simulink model "lab2"  (R2024a)
settings: Solver=FixedStepAuto  StartTime=0.0  StopTime=10.0  FixedStep=0.01  RelTol=1e-3
settings Model: Creator=ventus  LastModifiedBy=ventus

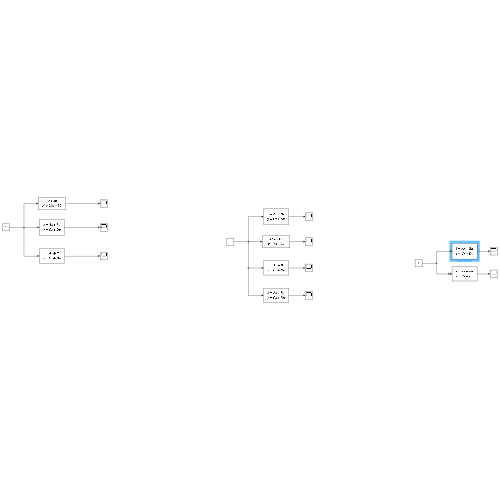
[thumbnail: Simulink's stored preview of the top-level diagram]
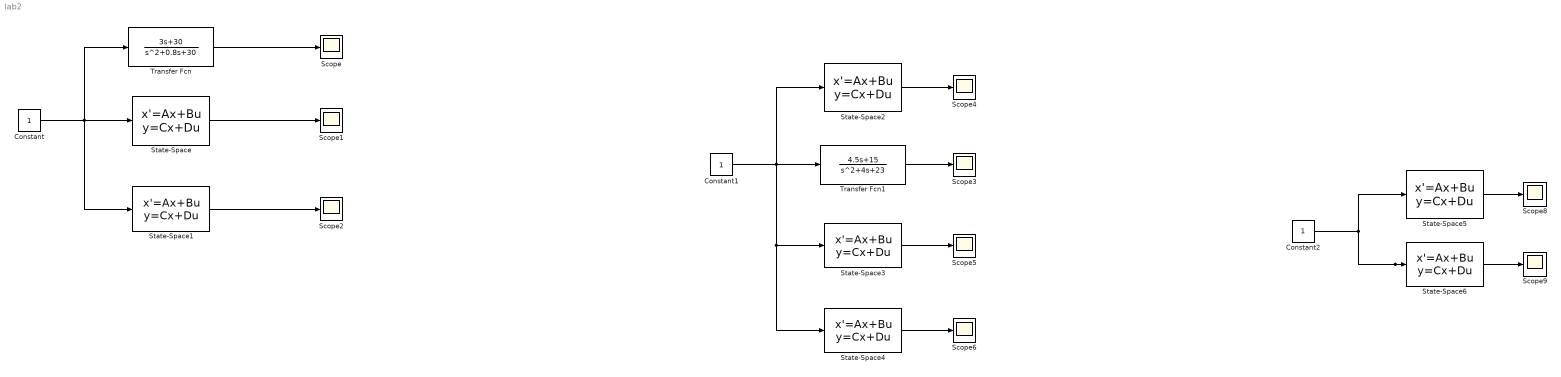
== system lab2 ==
  Constant : Constant
  Constant1 : Constant
  Constant2 : Constant
  Scope{,1..6,8..9} (9 alike) : Scope
  State-Space : StateSpace  A=[0 1; -30 -0.8]  B=[0; 1]  C=[30 3]  D=0  InitialCondition=0
  State-Space1 : StateSpace  A=[0 -30; 1 -0.8]  B=[30; 3]  C=[0 1]  D=0  InitialCondition=0
  State-Space2 : StateSpace  A=[-1 2; -10 -3]  B=[0.5; 1]  C=[6 1.5]  D=0  InitialCondition=0
  State-Space3 : StateSpace  A=[0 1; -23 -4]  B=[0; 1]  C=[15 4.5]  D=0  InitialCondition=0
  State-Space4 : StateSpace  A=[0 -23; 1 -4]  B=[15; 4.5]  C=[0 1]  D=0  InitialCondition=0
  State-Space5 : StateSpace  A=[-1 2; -10 -3]  B=[0.5; 1]  C=[6.5 1.5]  D=0  InitialCondition=0
  State-Space6 : StateSpace  A=[9 28; -5 -13]  B=[-0.5; 0.5]  C=[6.5 16]  D=0  InitialCondition=0
  Transfer Fcn : TransferFcn  Numerator=[3 30]  Denominator=[1 0.8 30]
  Transfer Fcn1 : TransferFcn  Numerator=[4.5 15]  Denominator=[1 4 23]
  wires:
  Constant/1 -> Transfer Fcn/1, State-Space/1, State-Space1/1
  State-Space/1 -> Scope1/1
  Transfer Fcn/1 -> Scope/1
  State-Space1/1 -> Scope2/1
  State-Space3/1 -> Scope5/1
  Transfer Fcn1/1 -> Scope3/1
  Constant1/1 -> State-Space4/1, State-Space3/1, State-Space2/1, Transfer Fcn1/1
  State-Space2/1 -> Scope4/1
  State-Space4/1 -> Scope6/1
  State-Space5/1 -> Scope8/1
  Constant2/1 -> State-Space6/1, State-Space5/1
  State-Space6/1 -> Scope9/1
